simulink model "Simulink_EMPS_Rigide"  (R2016b)
settings: Solver=ode23tb  StartTime=0.0  StopTime=10.0  FixedStep=tec  RelTol=1e-3  EnableMultiTasking=on
values from neighbouring files (symbols this model uses):
  filterq1 = [0.5000 0.5000]    [Simulation_EMPS.m]    (also in Simulation_EMPS_Validation.m)
  Fv1 = 203.5034    [Simulation_EMPS.m]    (also in Simulation_EMPS_Validation.m)
  gtau = 35.1506518825    [DATA_EMPS.mat]    (also in DATA_EMPS_PULSES.mat)
  kp = 160.18    [DATA_EMPS.mat]    (also in DATA_EMPS_PULSES.mat)
  kv = 243.45    [DATA_EMPS.mat]    (also in DATA_EMPS_PULSES.mat)
  M1 = 95.1089    [Simulation_EMPS.m]    (also in Simulation_EMPS_Validation.m)
  OF1 = -3.1648    [Simulation_EMPS.m]    (also in Simulation_EMPS_Validation.m)
  tec = t(10)-t(9)    [Simulation_EMPS.m]    (also in Simulation_EMPS_Validation.m)
  viradm = 10    [Simulation_EMPS.m]    (also in Simulation_EMPS_Validation.m)
libraries: simulink x2
settings Model: Creator=tony  LastModifiedBy=ajanot
settings DataIOCC: LimitDataPoints=on  SaveFormat=Array  SignalLoggingSaveFormat=ModelDataLogs
settings OptimizationCC: ExpressionDepthLimit=2147483647  InitFltsAndDblsToZero=on  LifeSpan=inf
settings DebuggingCC: UnderspecifiedInitializationDetection=Classic  MergeDetectMultiDrivingBlocksExec=none  SolverPrmCheckMsg=warning  FcnCallInpInsideContextMsg=warning  StateNameClashWarn=warning  SFUnexpectedBacktrackingDiag=warning  SFNoUnconditionalDefaultTransitionDiag=warning  SFExecutionAtInitializationDiag=none
settings HardwareCC: ProdBitPerPointer=32  ProdBitPerSizeT=32  ProdBitPerPtrDiffT=32  ProdLargestAtomicFloat=None  ProdIntDivRoundTo=Undefined  ProdEndianess=Unspecified  ProdWordSize=32  ProdHWDeviceType=32-bit Generic
settings ModelReferenceCC: PropagateSignalLabelsOutOfModel=off
settings GRTTargetCC: TargetLangStandard=C89/C90 (ANSI)  CombineOutputUpdateFcns=off  GRTInterface=on
settings ConfigComp: CovMetricSettings=dw  CovHtmlReporting=on  CovSaveCumulativeToWorkspaceVar=on  CovSaveSingleToWorkspaceVar=on  CovExternalEMLEnable=off

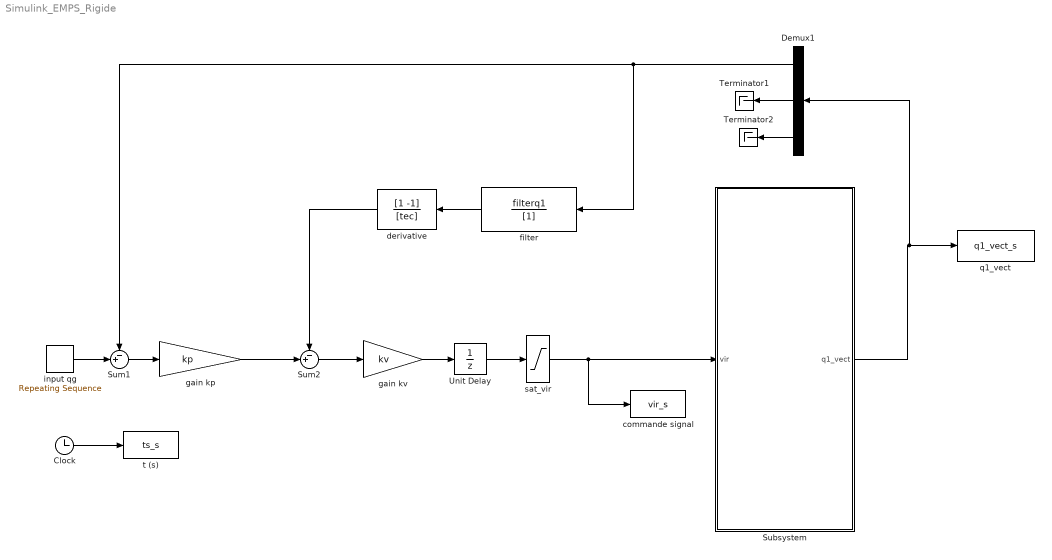
== system Simulink_EMPS_Rigide ==
  Clock : Clock
  Demux1 : Demux  Outputs=3
  Subsystem : Subsystem
  Sum1 : Sum  Inputs=-+|
  Sum2 : Sum  Inputs=-+|
  Terminator1 : Terminator
  Terminator2 : Terminator
  Unit Delay : UnitDelay  SampleTime=tec
  commande signal : ToWorkspace  VariableName=vir_s  SampleTime=tec
  derivative : DiscreteFilter  Numerator=[1 -1]  Denominator=[tec]  SampleTime=tec
  filter : DiscreteFilter  Numerator=filterq1  Denominator=[1]  SampleTime=tec
  gain kp : Gain  Gain=kp
  gain kv : Gain  Gain=kv
  input qg : simulink/Sources/Repeating Sequence  rep_seq_t=t  rep_seq_y=qg
  q1_vect : ToWorkspace  VariableName=q1_vect_s  SampleTime=tec
  sat_vir : Saturate  UpperLimit=viradm  LowerLimit=-viradm
  t (s) : ToWorkspace  VariableName=ts_s  SampleTime=tec
  wires:
  gain kv/1 -> Unit Delay/1
  Sum1/1 -> gain kp/1
  gain kp/1 -> Sum2/2
  Sum2/1 -> gain kv/1
  input qg/1 -> Sum1/2
  Unit Delay/1 -> sat_vir/1
  Clock/1 -> t (s)/1
  derivative/1 -> Sum2/1
  filter/1 -> derivative/1
  Subsystem/1(q1_vect) -> Demux1/1, q1_vect/1
  sat_vir/1 -> commande signal/1, Subsystem/1(vir)
  Demux1/2 -> Terminator1/1
  Demux1/3 -> Terminator2/1
  Demux1/1 -> filter/1, Sum1/1

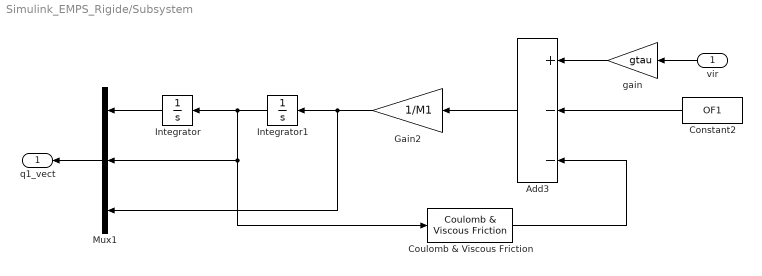
== system Simulink_EMPS_Rigide/Subsystem ==
  vir : Inport
  Add3 : Sum  Inputs=+--
  Constant2 : Constant  Value=OF1
  Coulomb & Viscous Friction : simulink/Discontinuities/Coulomb & Viscous Friction  offset=Fc1  gain=Fv1
  Gain2 : Gain  Gain=1/M1
  Integrator : Integrator
  Integrator1 : Integrator
  Mux1 : Mux  Inputs=3
  "gain " : Gain  Gain=gtau
  q1_vect : Outport
  wires:
  Add3/1 -> Gain2/1
  Gain2/1 -> Integrator1/1, Mux1/3
  Integrator1/1 -> Integrator/1, Mux1/2, Coulomb & Viscous Friction/1
  vir/1 -> "gain "/1
  "gain "/1 -> Add3/1
  Mux1/1 -> q1_vect/1
  Integrator/1 -> Mux1/1
  Constant2/1 -> Add3/2
  Coulomb & Viscous Friction/1 -> Add3/3
